simulink model "VCMGCM1962020b_v2"  (R2020b)
settings: Solver=FixedStepDiscrete  StartTime=0.0  StopTime=10.0  FixedStep=0.005  RelTol=1e-3  EnableMultiTasking=on
PreLoadFcn:
  | try, model_open; catch, disp('Error occurred while executing model pre-load callback: model_open.m'); disp('Please assure that the MATLAB working directory is set to the model directory before opening.'); end
InitFcn:
  | try, model_open; catch, end
undefined symbols (not defined in the file): Bridge, GCM, H, raptor_get_param_eval, raptor_get_safe_string, raptor_xcp_function
libraries: Blocks_lib x1165, Raptor_lib x665, simulink x62, VCM_lib x5
(part 20 of 23)

== system VCMGCM1962020b_v2/Fgnd/Virtual Sensors/Vehicle/Range/RangeGain/Subsystem ==
  y : Inport
  Enable : EnablePort
  Eqn(w/DvdByZeroPro) : Blocks_lib/Eqn(w//DvdByZeroPro)  eqn='u(1) / u(2)'  dmn='u(2)'  dfltval=0
  Out1 : Outport
  wires:
  y/1 -> Eqn(w/DvdByZeroPro)/1
  Eqn(w/DvdByZeroPro)/1 -> Out1/1

== system VCMGCM1962020b_v2/Fgnd/Actuators/CAN/Battery/ChgrBatt_State_Transition_Cmd/MsgTx/doublestrike ==
  note: Because of issues with the Romeo BMS this logic can be set up to apply main contactors followed by a reset and then contactor apply a second time
  <MainCntrReq [Bool]> : Inport
  AND{,2..4} (4 alike) : Logic  Operator=OR  AllPortsSameDT=off  OutDataTypeStr=boolean
  AND1 : Logic  AllPortsSameDT=off  OutDataTypeStr=boolean
  AND5 : Logic  AllPortsSameDT=off  OutDataTypeStr=boolean
  CntrSat1 : Blocks_lib/CntrSat  init=0  inc=1  typ=uint8  relop=>=  th_nam='MaincntrTurnOn'  th_gain=samptime  th_units='sec'  th_help='Counter threshold'  th_group='Group'
  CntrSat2 : Blocks_lib/CntrSat  init=0  inc=1  typ=uint8  relop=>=  th_nam='MaincntrTurnOff'  th_gain=samptime  th_units='sec'  th_help='Counter threshold'  th_group='Group'
  Falling edge : Subsystem
  Header : Blocks_lib/Header  width=Landscape  addtext=''
  NOT : Logic  Operator=NOT  AllPortsSameDT=off  OutDataTypeStr=boolean
  NOT1 : Logic  Operator=NOT  AllPortsSameDT=off  OutDataTypeStr=boolean
  raptor_adjustment : Raptor_lib/Data Storage/raptor_adjustment  paramName='RomoBMS2Strike'  nameSource=Parameter  initValue=0  dataType=boolean  storage=Calibration  calDispType=Number  calEnum={'False', 'True'}  calGain=1.0  calOffset=0.0  calMax=inf  calMin=-inf  calFormat='-1'  calUnit='Bool'  calHelp=' set this to 1 to turn on Batt main contr double strike logic'  calAccess=1  calFunction='Actuator | Batt '  calDispHeaders=off  calColHeaders={'Col1' 'Col2' 'Col3'}  calRowHeaders={'Row1' 'Row2' 'Row3'}
      settings: SourceProductName=Raptor
  raptor_measurement : Raptor_lib/Data Storage/raptor_measurement  paramName='CntrTest1'  nameSource=Parameter  calDispType=Number  calEnum={'False', 'True'}  calGain=1.0  calOffset=0.0  calMax=inf  calMin=-inf  calFormat='-1'  calUnit='bool'  calHelp='contactor reset logic test'  calAccess=1  calFunction=' Actuator | BMSTest'  calVisible=on
      settings: SourceProductName=Raptor
  raptor_measurement1 : Raptor_lib/Data Storage/raptor_measurement  paramName='CntrTest2'  nameSource=Parameter  calDispType=Number  calEnum={'False', 'True'}  calGain=1.0  calOffset=0.0  calMax=inf  calMin=-inf  calFormat='-1'  calUnit='bool'  calHelp='contactor reset logic test'  calAccess=1  calFunction=' Actuator | BMSTest'  calVisible=on
      settings: SourceProductName=Raptor
  rising edge : Subsystem
  rising edge1 : Subsystem
  HiVolt_Bus_Connect_Cmd1 : Outport
  wires:
  <MainCntrReq [Bool]>/1 -> CntrSat2/1, AND5/1, AND1/2, Falling edge/1(In), rising edge/1(In)
  AND3/1 -> CntrSat1/2
  AND1/1 -> AND/2
  NOT/1 -> AND1/1
  rising edge/1(rising) -> AND2/1
  CntrSat1/1 -> AND/1, raptor_measurement1/1
  Falling edge/1(falling) -> AND3/2, AND2/2
  CntrSat2/1 -> rising edge1/1(In), NOT/1, raptor_measurement/1, CntrSat1/1
  rising edge1/1(rising) -> AND3/1
  AND2/1 -> CntrSat2/2
  AND4/1 -> HiVolt_Bus_Connect_Cmd1/1
  AND/1 -> AND4/1  "HiVolt_Bus_Connect_Cmd"
  AND5/1 -> AND4/2
  raptor_adjustment/1 -> NOT1/1
  NOT1/1 -> AND5/2

== system VCMGCM1962020b_v2/Fgnd/Actuators/CAN/CCS Interface/CCSEV_ChargeParameters1/MsgTx/EVEnergyRequest ==
  Data : Inport
  Bus Selector : BusSelector  OutputSignals=VirtualSensors.Batt.BattSOC [%]
  Fcn : Fcn  Expr=u(1) * (u(2) - u(3)) /100
  Header : Blocks_lib/Header  width=Portrait  addtext=''
  Meas&Ovrd : Blocks_lib/Meas&Ovrd  nam=[nam 'EVEnergyRequest']  name_source=Parameter  view_as=Number  enum_struct={}  gain=1  min=-inf  max=inf  precision=''  units='kWh'  help='CAN message value'  group=['Actuators | CAN | ' msgnam]
  Mux : Mux  Inputs=3
  raptor_data_read : Raptor_lib/Data Storage/raptor_data_read  dataName=[nam 'FullSOC']  dataShape=Scalar  idxSource=Input  idxRow=1  idxCol=1
      settings: SourceProductName=Raptor
  raptor_data_read2 : Raptor_lib/Data Storage/raptor_data_read  dataName=[nam 'EnergyCapacity']  dataShape=Scalar  idxSource=Input  idxRow=1  idxCol=1
      settings: SourceProductName=Raptor
  kWh : Outport  VectorParamsAs1DForOutWhenUnconnected=off
  wires:
  Fcn/1 -> Meas&Ovrd/1
  Meas&Ovrd/1 -> kWh/1
  Bus Selector/1 -> Mux/3  "<BattSOC [%]>"
  Mux/1 -> Fcn/1
  raptor_data_read2/1 -> Mux/1
  raptor_data_read/1 -> Mux/2
  Data/1 -> Bus Selector/1

== system VCMGCM1962020b_v2/Fgnd/Actuators/CAN/CCS Interface/CCSEV_DC_ChargeInfo1/MsgTx/RemainingTime ==
  Data : Inport
  Bus Selector : BusSelector  OutputSignals=VirtualSensors.Batt.BattSOC [%],VirtualSensors.Batt.BattVolt [V],VirtualSensors.Batt.BattCur [A]
  Compare To Zero : simulink/Logic and Bit Operations/Compare To Zero  relop=<=  OutDataTypeStr=boolean
  Constant : Constant  Value=double(0)
  Demux : Demux  Outputs=2
  Eqn(w/DvdByZeroPro) : Blocks_lib/Eqn(w//DvdByZeroPro)  eqn='- u(1) * (u(2) - u(4)) / (u(5) * u(6)) * 600'  dmn='(u(5) * u(6))'  dfltval=127.5
  Eqn(w/DvdByZeroPro)1 : Blocks_lib/Eqn(w//DvdByZeroPro)  eqn='- u(1) * (u(3) - u(4)) / (u(5) * u(6)) * 600'  dmn='(u(5) * u(6))'  dfltval=127.5
  Fcn : Fcn  Expr=u(2) - u(4)
  Fcn1 : Fcn  Expr=u(3) - u(4)
  Filt : Blocks_lib/Filt  nam=[nam 'RemainingTimeFiltTC']  group=['Actuators | CAN | ' msgnam]  samptime=samptime
  Header : Blocks_lib/Header  width=Portrait  addtext=''
  Meas&Ovrd : Blocks_lib/Meas&Ovrd  nam=[nam 'RemainingTimeToFullSOC']  name_source=Parameter  view_as=Number  enum_struct={}  gain=1  min=-inf  max=inf  precision=''  units='minutes'  help='CAN message value'  group=['Actuators | CAN | ' msgnam]
  Meas&Ovrd1 : Blocks_lib/Meas&Ovrd  nam=[nam 'RemainingTimeToBulkSOC']  name_source=Parameter  view_as=Number  enum_struct={}  gain=1  min=-inf  max=inf  precision=''  units='minutes'  help='CAN message value'  group=['Actuators | CAN | ' msgnam]
  Multiport Switch : MultiPortSwitch  DataPortOrder=Zero-based contiguous  Inputs=2  zeroidx=on
  Mux : Mux  Inputs=6
  Mux1 : Mux  Inputs=2
  Mux2 : Mux  Inputs=2
  Saturation : Saturate  UpperLimit=0  LowerLimit=-inf
  Saturation1 : Saturate  UpperLimit=127.5  LowerLimit=0
  raptor_data_read : Raptor_lib/Data Storage/raptor_data_read  dataName=[nam 'FullSOC']  dataShape=Scalar  idxSource=Input  idxRow=1  idxCol=1
      settings: SourceProductName=Raptor
  raptor_data_read1 : Raptor_lib/Data Storage/raptor_data_read  dataName=[nam 'BulkSOC']  dataShape=Scalar  idxSource=Input  idxRow=1  idxCol=1
      settings: SourceProductName=Raptor
  raptor_data_read2 : Raptor_lib/Data Storage/raptor_data_read  dataName=[nam 'EnergyCapacity']  dataShape=Scalar  idxSource=Input  idxRow=1  idxCol=1
      settings: SourceProductName=Raptor
  Full : Outport  VectorParamsAs1DForOutWhenUnconnected=off
  Bulk : Outport  Port=2  VectorParamsAs1DForOutWhenUnconnected=off
  wires:
  Mux/1 -> Eqn(w/DvdByZeroPro)1/1, Eqn(w/DvdByZeroPro)/1, Fcn1/1, Fcn/1
  raptor_data_read1/1 -> Mux/3
  raptor_data_read/1 -> Mux/2
  Bus Selector/3 -> Saturation/1  "<BattCur [A]>"
  Bus Selector/2 -> Mux/5  "<BattVolt [V]>"
  Bus Selector/1 -> Mux/4  "<BattSOC [%]>"
  Meas&Ovrd1/1 -> Bulk/1
  raptor_data_read2/1 -> Mux/1
  Data/1 -> Bus Selector/1
  Meas&Ovrd/1 -> Full/1
  Saturation/1 -> Mux/6
  Eqn(w/DvdByZeroPro)/1 -> Mux1/1
  Eqn(w/DvdByZeroPro)1/1 -> Mux1/2
  Fcn/1 -> Mux2/1
  Fcn1/1 -> Mux2/2
  Mux2/1 -> Compare To Zero/1
  Compare To Zero/1 -> Multiport Switch/1
  Mux1/1 -> Multiport Switch/2
  Constant/1 -> Multiport Switch/3
  Saturation1/1 -> Filt/1
  Demux/1 -> Meas&Ovrd/1
  Demux/2 -> Meas&Ovrd1/1
  Filt/1 -> Demux/1
  Multiport Switch/1 -> Saturation1/1

== system VCMGCM1962020b_v2/Fgnd/Actuators/CAN/CCS Interface/Commands/Charge Port DC Voltage Diag/EvalDiag ==
  Data : Inport
  Reset : EnablePort  StatesWhenEnabling=reset
  Bus Selector : BusSelector  OutputSignals=VirtualSensors.Chgr.ChgPortDCVolt [V]
  FltRngTmr : Blocks_lib/FltRngTmr  nam='ChgPortDCVoltHi'  relop=>  threshnam='ChgPortDCVoltHiThr'  typ=double  units='V'  help='Range high fault threshold'  tmrth_nam='ChgPortDCVoltHiTimeThr'  tmrth_typ=uint16  tmrth_help='Range high fault time threshold'  samptime=samptime  group='Diagnostics | System'
  Header : Blocks_lib/Header  width=Portrait  addtext=''
  wires:
  Bus Selector/1 -> FltRngTmr/1  "<ChgPortDCVolt [V]>"
  Data/1 -> Bus Selector/1

== system VCMGCM1962020b_v2/Fgnd/Actuators/CAN/Charger/Config Msgs/Config Sequence/0x616 ==
  f : TriggerPort  TriggerType=function-call  VariantControl=Variant  PortDimensions=1
  Constant : Constant  Value=uint8(hex2dec('A5'))
  Header : Blocks_lib/Header  width=Portrait  addtext=''
  Logical Operator : Logic  Inputs=1  AllPortsSameDT=off  OutDataTypeStr=boolean
  Mux : Mux  Inputs=2
  Relational Operator : RelationalOperator  Operator===  OutDataTypeStr=boolean  RndMeth=Simplest
  Terminator : Terminator
  Terminator1 : Terminator
  Terminator2 : Terminator
  raptor_adjustment : Raptor_lib/Data Storage/raptor_adjustment  paramName='ChgrConfigData'  nameSource=Parameter  initValue=zeros(1,7)  dataType=uint8  storage=Calibration  calDispType=Number  calEnum={'False', 'True'}  calGain=1  calOffset=0  calMax=inf  calMin=-inf  calFormat=''  calUnit=''  calHelp='Charger configuration data'  calAccess=1  calFunction='Actuators | CAN | ChgrConfig'  calDispHeaders=off  calColHeaders={'Col1' 'Col2' 'Col3'}  calRowHeaders={'Row1' 'Row2' 'Row3'}
      settings: SourceProductName=Raptor
  raptor_can_rxraw : Raptor_lib/CAN/raptor_can_rxraw  canBus=bus  extendedId=0  showAge=0  id=hex2dec('616')  idMask=hex2dec('7FF')  mailbox='Chgr616Msg'  queueSize=1
      settings: SourceProductName=Raptor
  raptor_data_def : Raptor_lib/Data Storage/raptor_data_def  dataName='ChgrConfigComplete'  initValue=0  dataType=boolean  storage=Volatile (RAM)  calVisible=on  calType=Measurement  calDispType=Number  calEnum={'False', 'True'}  calGain=1.0  calOffset=0  calMin=-inf  calMax=inf  calFormat='-1'  calUnit='Bool'  calHelp='Charger configuration complete'  calAccess=1  calFunction='Actuators | CAN | ChgrConfig'  calDispHeaders=off  calColHeaders={'Col1' 'Col2' 'Col3'}  calRowHeaders={'Row1' 'Row2' 'Row3'}
      settings: SourceProductName=Raptor
  raptor_data_write : Raptor_lib/Data Storage/raptor_data_write  dataName='ChgrConfigComplete'  dataShape=Scalar  idxSource=Input Port  idxRow=1  idxCol=1
      settings: SourceProductName=Raptor
  wires:
  raptor_can_rxraw/1 -> Terminator/1
  raptor_can_rxraw/2 -> Terminator1/1
  raptor_can_rxraw/3 -> Terminator2/1
  raptor_can_rxraw/4 -> Relational Operator/1
  Logical Operator/1 -> raptor_data_write/1
  raptor_adjustment/1 -> Mux/1
  Constant/1 -> Mux/2
  Mux/1 -> Relational Operator/2
  Relational Operator/1 -> Logical Operator/1

== system VCMGCM1962020b_v2/Fgnd/Actuators/CAN/Charger/Config Msgs/Config Sequence/0x617_00 ==
  f : TriggerPort  TriggerType=function-call  VariantControl=Variant  PortDimensions=1
  Constant : Constant  Value=boolean(0)
  Constant1 : Constant  Value=uint32(hex2dec('617'))
  Constant2 : Constant  Value=uint8(8)
  Constant4 : Constant  Value=uint8(hex2dec('00'))
  Header : Blocks_lib/Header  width=Portrait  addtext=''
  Mux : Mux  Inputs=2
  raptor_can_txraw : Raptor_lib/CAN/raptor_can_txraw  canBus=bus  queueSize=1  showIdTypePort=1  idTypeSelectValues=Standard|Extended  idTypeSelect=Standard
      settings: SourceProductName=Raptor
  raptor_data_read : Raptor_lib/Data Storage/raptor_data_read  dataName='ChgrConfigData'  dataShape=Vector  idxSource=Read Entire Vector/Matrix  idxRow=1  idxCol=1
      settings: SourceProductName=Raptor
  wires:
  Constant2/1 -> raptor_can_txraw/3
  Constant1/1 -> raptor_can_txraw/2
  Constant/1 -> raptor_can_txraw/1
  Constant4/1 -> Mux/2
  raptor_data_read/1 -> Mux/1
  Mux/1 -> raptor_can_txraw/4

== system VCMGCM1962020b_v2/Fgnd/Actuators/CAN/Charger/Config Msgs/Config Sequence/0x617_A5 ==
  f : TriggerPort  TriggerType=function-call  VariantControl=Variant  PortDimensions=1
  Constant : Constant  Value=boolean(0)
  Constant1 : Constant  Value=uint32(hex2dec('617'))
  Constant2 : Constant  Value=uint8(8)
  Constant4 : Constant  Value=uint8(hex2dec('A5'))
  Header : Blocks_lib/Header  width=Portrait  addtext=''
  Mux : Mux  Inputs=2
  raptor_can_txraw : Raptor_lib/CAN/raptor_can_txraw  canBus=bus  queueSize=1  showIdTypePort=1  idTypeSelectValues=Standard|Extended  idTypeSelect=Standard
      settings: SourceProductName=Raptor
  raptor_data_read : Raptor_lib/Data Storage/raptor_data_read  dataName='ChgrConfigData'  dataShape=Vector  idxSource=Read Entire Vector/Matrix  idxRow=1  idxCol=1
      settings: SourceProductName=Raptor
  wires:
  Constant/1 -> raptor_can_txraw/1
  Constant1/1 -> raptor_can_txraw/2
  Constant2/1 -> raptor_can_txraw/3
  Mux/1 -> raptor_can_txraw/4
  Constant4/1 -> Mux/2
  raptor_data_read/1 -> Mux/1

== system VCMGCM1962020b_v2/Fgnd/Actuators/CAN/Drive Inverter/NMT Trasition Command/Inverter Error Reset/rising edge2 ==
  <RunMode [Bool]> : Inport
  AND6 : Logic  AllPortsSameDT=off  OutDataTypeStr=boolean
  NOT1 : Logic  Operator=NOT  AllPortsSameDT=off  OutDataTypeStr=boolean
  Unit Delay : UnitDelay  SampleTime=-1  HasFrameUpgradeWarning=on
  rising : Outport
  wires:
  Unit Delay/1 -> AND6/1
  NOT1/1 -> AND6/2
  AND6/1 -> rising/1
  <RunMode [Bool]>/1 -> NOT1/1, Unit Delay/1

== system VCMGCM1962020b_v2/Fgnd/Actuators/CAN/Other/A//C Compressor/MsgName/MsgTx ==
  Data : Inport
  Enable : EnablePort
  Bus Selector : BusSelector  OutputSignals=Control.Other.ACC.ACCSpdReq [rpm],Sensors.Sensors.Volt.DRVPVolt.DRVPVolt [V]
  CANTxField : Blocks_lib/CANTxField  custom=on  custom_nam=[nam '---']  custom_units='---'
  CANTxField1 : Blocks_lib/CANTxField  custom=on  custom_nam=[nam '---']  custom_units='---'
  Header : Blocks_lib/Header  width=Landscape  addtext=''
  Key Start : Subsystem
  raptor_can_txmsg : Raptor_lib/CAN/raptor_can_txmsg  canDefinition=struct('dbcFile', 'ACCompressor_MitsubishiEV36BNx.dbc','message', 'REQ','comment', '','signals', {{'SpdReq','BATT_VOLT','KeyStart'}},'enabled', [ 1 1 1;],'scaled', [ 1 1 1;],'canBus', 'bus','messageID', [ 202154048;],'idMask', [ 536870911;],'payloadMask', [],'payloadValue', [],'period', [ 100;],'mailbox', '''''','queueSize', [ 1;],'label', [ 1;],'ver', [ 2;],'showID', [ 0;],'showRaw', [ 0;],'fill', [ 1;],'editID', [ 0;],'signalOrder', [ 3;],'signalAscDes', [ 1;])  canBus=bus  queueSize=1  payloadMask=[]  payloadValue=[]  period=100  showID=0  label=1  idMask=hex2dec('1FFFFFFF')  fill=1  id=202154048  showRaw=0  signalOrder=3  signalInfo={{struct('Name', 'SpdReq','Startbit', [ 0;],'SignalSize', [ 14;],'ByteOrder', 'BigEndian','ValueType', 'UNSIGNED','Class', 'uint16','Signed', [ 0;],'Factor', [ 1;],'Offset', [ 0;],'Min', [ 960;],'Max', [ 8640;],'Units', 'RPM','Comment', '','StartBit', [ 8;]),struct('Name', 'BATT_VOLT','Startbit', [ 0;],'SignalSize', [ 8;],'ByteOrder', 'LittleEndian','ValueType', 'UNSIGNED','Class', 'uint8','Signed', [ 0;],'Factor', [ 0.1;],'Offset', [ 0;],'Min', [ 0;],'Max', [ 25.5;],'Units', 'Volts','Comment', '','StartBit', [ 24;]),struct('Name', 'KeyStart','Startbit', [ 0;],'SignalSize', [ 4;],'ByteOrder', 'LittleEndian','ValueType', 'UNSIGNED','Class', 'uint8','Signed', [ 0;],'Factor', [ 1;],'Offset', [ 0;],'Min', [ 0;],'Max', [ 3;],'Units', '','Comment', '','StartBit', [ 36;])}}
      settings: SourceProductName=Raptor
  wires:
  Data/1 -> Key Start/1(Data), Bus Selector/1
  CANTxField1/1 -> raptor_can_txmsg/2  "BATT_VOLT"
  Bus Selector/2 -> CANTxField1/1  "<DRVPVolt [V]>"
  Key Start/1(enum) -> raptor_can_txmsg/3  "KeyStart"
  CANTxField/1 -> raptor_can_txmsg/1  "SpdReq"
  Bus Selector/1 -> CANTxField/1  "<ACCSpdReq [rpm]>"

== system VCMGCM1962020b_v2/Fgnd/Actuators/CAN/Other/Cooling Pump 1/MsgName/MsgTx ==
  Data : Inport
  Enable : EnablePort
  Bus Selector : BusSelector  OutputSignals=Control.Other.CoolPump.CoolPump1EnblReq [Bool]
  Bus Selector1 : BusSelector  OutputSignals=Control.Other.CoolPump.CoolPump1SpdReq [%]
  CANTxField : Blocks_lib/CANTxField  custom=on  custom_nam=[nam '---']  custom_units='---'
  CANTxField1 : Blocks_lib/CANTxField  custom=on  custom_nam=[nam '---']  custom_units='---'
  Data Type Conversion : DataTypeConversion  OutDataTypeStr=uint32
  Header : Blocks_lib/Header  width=Landscape  addtext=''
  Shift Arithmetic : ArithShift  BitShiftNumber=-8
  raptor_adjustment : Raptor_lib/Data Storage/raptor_adjustment  paramName=[nam 'PowerHold']  nameSource=Parameter  initValue=0.00  dataType=uint8  storage=Calibration  calDispType=Number  calEnum={'False', 'True'}  calGain=1.0  calOffset=0.0  calMax=inf  calMin=-inf  calFormat='-1'  calUnit=''  calHelp='Power hold'  calAccess=1  calFunction=['Actuators | CAN | ' msgnam]  calDispHeaders=off  calColHeaders={'Col1' 'Col2' 'Col3'}  calRowHeaders={'Row1' 'Row2' 'Row3'}
      settings: SourceProductName=Raptor
  raptor_can_txmsg : Raptor_lib/CAN/raptor_can_txmsg  canDefinition=struct('dbcFile', 'EMPMotorController.dbc','message', 'EAPMCPC','comment', '','signals', {{'EnableCommand','PowerHold','SpeedCommand','PercentSpeed'}},'enabled', [ 1 1 1 0;],'canBus', 'bus','messageID', [ 410648576;],'idMask', [ 536805631;],'payloadMask', [],'payloadValue', [],'period', [ 1000;],'mailbox', '''''','queueSize', [ 1;],'label', [ 1;],'ver', [ 2;],'showID', [ 1;],'showRaw', [ 0;],'fill', [ 1;],'editID', [ 0;],'signalOrder', [ 3;])  canBus=bus  queueSize=1  payloadMask=[]  payloadValue=[]  period=1000  showID=1  label=1  idMask=hex2dec('1FFF00FF')  fill=1  id=410648576  showRaw=0  signalOrder=3  signalInfo={{struct('Name', 'EnableCommand','Startbit', [ 0;],'SignalSize', [ 2;],'ByteOrder', 'LittleEndian','ValueType', 'UNSIGNED','Class', 'uint8','Signed', [ 0;],'Factor', [ 1;],'Offset', [ 0;],'Min', [ 0;],'Max', [ 3;],'Units', '','Comment', '','StartBit', [ 0;]),struct('Name', 'PowerHold','Startbit', [ 0;],'SignalSize', [ 2;],'ByteOrder', 'LittleEndian','ValueType', 'UNSIGNED','Class', 'uint8','Signed', [ 0;],'Factor', [ 1;],'Offset', [ 0;],'Min', [ 0;],'Max', [ 3;],'Units', '','Comment', '','StartBit', [ 2;]),struct('Name', 'SpeedCommand','Startbit', [ 0;],'SignalSize', [ 16;],'ByteOrder', 'LittleEndian','ValueType', 'UNSIGNED','Class', 'uint16','Signed', [ 0;],'Factor', [ 0.5;],'Offset', [ 0;],'Min', [ 0;],'Max', [ 32127.5;],'Units', 'rpm','Comment', '','StartBit', [ 8;]),struct('Name', 'PercentSpeed','Startbit', [ 0;],'SignalSize', [ 8;],'ByteOrder', 'LittleEndian','ValueType', 'UNSIGNED','Class', 'uint8','Signed', [ 0;],'Factor', [ 0.5;],'Offset', [ 0;],'Min', [ 0;],'Max', [ 125;],'Units', '%','Comment', '','StartBit', [ 24;])}}
      settings: SourceProductName=Raptor
  raptor_data_read : Raptor_lib/Data Storage/raptor_data_read  dataName=[nam 'J1939SA']  dataShape=Scalar  idxSource=Input  idxRow=1  idxCol=1
      settings: SourceProductName=Raptor
  wires:
  Shift Arithmetic/1 -> raptor_can_txmsg/1
  raptor_data_read/1 -> Data Type Conversion/1
  Data Type Conversion/1 -> Shift Arithmetic/1
  raptor_adjustment/1 -> raptor_can_txmsg/3  "PowerHold"
  CANTxField1/1 -> raptor_can_txmsg/4  "SpeedCommand"
  Bus Selector1/1 -> CANTxField1/1  "<CoolPump1SpdReq [%]>"
  Bus Selector/1 -> CANTxField/1  "<CoolPump1EnblReq [Bool]>"
  CANTxField/1 -> raptor_can_txmsg/2  "EnableCommand"
  Data/1 -> Bus Selector/1, Bus Selector1/1

== system VCMGCM1962020b_v2/Fgnd/Actuators/CAN/Other/Cooling Pump 2/MsgName/MsgTx ==
  Data : Inport
  Enable : EnablePort
  Bus Selector : BusSelector  OutputSignals=Control.Other.CoolPump.CoolPump2EnblReq [Bool]
  Bus Selector1 : BusSelector  OutputSignals=Control.Other.CoolPump.CoolPump2SpdReq [%]
  CANTxField : Blocks_lib/CANTxField  custom=on  custom_nam=[nam '---']  custom_units='---'
  CANTxField1 : Blocks_lib/CANTxField  custom=on  custom_nam=[nam '---']  custom_units='---'
  Data Type Conversion : DataTypeConversion  OutDataTypeStr=uint32
  Header : Blocks_lib/Header  width=Landscape  addtext=''
  Shift Arithmetic : ArithShift  BitShiftNumber=-8
  raptor_adjustment : Raptor_lib/Data Storage/raptor_adjustment  paramName=[nam 'PowerHold']  nameSource=Parameter  initValue=0.00  dataType=uint8  storage=Calibration  calDispType=Number  calEnum={'False', 'True'}  calGain=1.0  calOffset=0.0  calMax=inf  calMin=-inf  calFormat='-1'  calUnit=''  calHelp='Power hold'  calAccess=1  calFunction=['Actuators | CAN | ' msgnam]  calDispHeaders=off  calColHeaders={'Col1' 'Col2' 'Col3'}  calRowHeaders={'Row1' 'Row2' 'Row3'}
      settings: SourceProductName=Raptor
  raptor_can_txmsg : Raptor_lib/CAN/raptor_can_txmsg  canDefinition=struct('dbcFile', 'EMPMotorController.dbc','message', 'EAPMCPC','comment', '','signals', {{'EnableCommand','PowerHold','SpeedCommand','PercentSpeed'}},'enabled', [ 1 1 1 0;],'canBus', 'bus','messageID', [ 410648576;],'idMask', [ 536805631;],'payloadMask', [],'payloadValue', [],'period', [ 1000;],'mailbox', '''''','queueSize', [ 1;],'label', [ 1;],'ver', [ 2;],'showID', [ 1;],'showRaw', [ 0;],'fill', [ 1;],'editID', [ 0;],'signalOrder', [ 3;])  canBus=bus  queueSize=1  payloadMask=[]  payloadValue=[]  period=1000  showID=1  label=1  idMask=hex2dec('1FFF00FF')  fill=1  id=410648576  showRaw=0  signalOrder=3  signalInfo={{struct('Name', 'EnableCommand','Startbit', [ 0;],'SignalSize', [ 2;],'ByteOrder', 'LittleEndian','ValueType', 'UNSIGNED','Class', 'uint8','Signed', [ 0;],'Factor', [ 1;],'Offset', [ 0;],'Min', [ 0;],'Max', [ 3;],'Units', '','Comment', '','StartBit', [ 0;]),struct('Name', 'PowerHold','Startbit', [ 0;],'SignalSize', [ 2;],'ByteOrder', 'LittleEndian','ValueType', 'UNSIGNED','Class', 'uint8','Signed', [ 0;],'Factor', [ 1;],'Offset', [ 0;],'Min', [ 0;],'Max', [ 3;],'Units', '','Comment', '','StartBit', [ 2;]),struct('Name', 'SpeedCommand','Startbit', [ 0;],'SignalSize', [ 16;],'ByteOrder', 'LittleEndian','ValueType', 'UNSIGNED','Class', 'uint16','Signed', [ 0;],'Factor', [ 0.5;],'Offset', [ 0;],'Min', [ 0;],'Max', [ 32127.5;],'Units', 'rpm','Comment', '','StartBit', [ 8;]),struct('Name', 'PercentSpeed','Startbit', [ 0;],'SignalSize', [ 8;],'ByteOrder', 'LittleEndian','ValueType', 'UNSIGNED','Class', 'uint8','Signed', [ 0;],'Factor', [ 0.5;],'Offset', [ 0;],'Min', [ 0;],'Max', [ 125;],'Units', '%','Comment', '','StartBit', [ 24;])}}
      settings: SourceProductName=Raptor
  raptor_data_read : Raptor_lib/Data Storage/raptor_data_read  dataName=[nam 'J1939SA']  dataShape=Scalar  idxSource=Input  idxRow=1  idxCol=1
      settings: SourceProductName=Raptor
  wires:
  Data/1 -> Bus Selector1/1, Bus Selector/1
  CANTxField/1 -> raptor_can_txmsg/2  "EnableCommand"
  Bus Selector/1 -> CANTxField/1  "<CoolPump2EnblReq [Bool]>"
  Bus Selector1/1 -> CANTxField1/1  "<CoolPump2SpdReq [%]>"
  CANTxField1/1 -> raptor_can_txmsg/4  "SpeedCommand"
  raptor_adjustment/1 -> raptor_can_txmsg/3  "PowerHold"
  Data Type Conversion/1 -> Shift Arithmetic/1
  raptor_data_read/1 -> Data Type Conversion/1
  Shift Arithmetic/1 -> raptor_can_txmsg/1

== system VCMGCM1962020b_v2/Fgnd/Actuators/CAN/Other/Heater/MsgName/MsgTx ==
  Data : Inport
  Enable : EnablePort
  Bus Selector : BusSelector  OutputSignals=Control.Other.Heater.HeaterOutletTempReq [degC]
  Bus Selector1 : BusSelector  OutputSignals=Control.Other.Heater.HeaterEnblReq [Bool]
  CANTxField : Blocks_lib/CANTxField  custom=off  custom_nam='---'  custom_units='---'
  CANTxField1 : Blocks_lib/CANTxField  custom=off  custom_nam='---'  custom_units='---'
  Header : Blocks_lib/Header  width=Landscape  addtext=''
  raptor_adjustment : Raptor_lib/Data Storage/raptor_adjustment  paramName='HTR_PWR_LIMIT'  nameSource=Parameter  initValue=0  dataType=double  storage=Calibration  calDispType=Number  calEnum={'False', 'True'}  calGain=1.0  calOffset=0.0  calMax=inf  calMin=-inf  calFormat='-1'  calUnit='W'  calHelp='Heater power limit'  calAccess=1  calFunction=['Actuators | CAN | ' msgnam]  calDispHeaders=off  calColHeaders={'Col1' 'Col2' 'Col3'}  calRowHeaders={'Row1' 'Row2' 'Row3'}
      settings: SourceProductName=Raptor
  raptor_adjustment1 : Raptor_lib/Data Storage/raptor_adjustment  paramName='ECU_MODE'  nameSource=Parameter  initValue=0  dataType=uint8  storage=Calibration  calDispType=Number  calEnum={'False', 'True'}  calGain=1.0  calOffset=0.0  calMax=inf  calMin=-inf  calFormat='-1'  calUnit=''  calHelp='ECU mode'  calAccess=1  calFunction=['Actuators | CAN | ' msgnam]  calDispHeaders=off  calColHeaders={'Col1' 'Col2' 'Col3'}  calRowHeaders={'Row1' 'Row2' 'Row3'}
      settings: SourceProductName=Raptor
  raptor_can_txmsg : Raptor_lib/CAN/raptor_can_txmsg  canDefinition=struct('dbcFile', 'ATSS17002_EWH40Dx-245.dbc','message', 'Data_Set_1','comment', '','signals', {{'HTR_OUTPUT_REQ','HTR_PWR_LIMIT','ECU_MODE','HTR_ENABLE'}},'enabled', [ 1 1 1 1;],'canBus', 'bus','messageID', [ 972;],'idMask', [ 536870911;],'payloadMask', [],'payloadValue', [],'period', [ 100;],'mailbox', '''''','queueSize', [ 1;],'label', [ 1;],'ver', [ 2;],'showID', [ 0;],'showRaw', [ 0;],'fill', [ 1;],'editID', [ 0;],'signalOrder', [ 3;])  canBus=bus  queueSize=1  payloadMask=[]  payloadValue=[]  period=100  showID=0  label=1  idMask=hex2dec('1FFFFFFF')  fill=1  id=972  showRaw=0  signalOrder=3  signalInfo={{struct('Name', 'HTR_OUTPUT_REQ','Startbit', [ 0;],'SignalSize', [ 8;],'ByteOrder', 'BigEndian','ValueType', 'UNSIGNED','Class', 'uint8','Signed', [ 0;],'Factor', [ 1;],'Offset', [ 0;],'Min', [ 0;],'Max', [ 80;],'Units', 'degC','Comment', 'Heater Output Request','StartBit', [ 0;]),struct('Name', 'HTR_PWR_LIMIT','Startbit', [ 0;],'SignalSize', [ 8;],'ByteOrder', 'BigEndian','ValueType', 'UNSIGNED','Class', 'uint8','Signed', [ 0;],'Factor', [ 40;],'Offset', [ 0;],'Min', [ 0;],'Max', [ 10160;],'Units', 'W','Comment', 'Heater Power Limit','StartBit', [ 8;]),struct('Name', 'ECU_MODE','Startbit', [ 0;],'SignalSize', [ 4;],'ByteOrder', 'BigEndian','ValueType', 'UNSIGNED','Class', 'uint8','Signed', [ 0;],'Factor', [ 1;],'Offset', [ 0;],'Min', [ 0;],'Max', [ 15;],'Units', '','Comment', 'Power Status Signal','StartBit', [ 16;]),struct('Name', 'HTR_ENABLE','Startbit', [ 0;],'SignalSize', [ 1;],'ByteOrder', 'BigEndian','ValueType', 'UNSIGNED','Class', 'uint8','Signed', [ 0;],'Factor', [ 1;],'Offset', [ 0;],'Min', [ 0;],'Max', [ 1;],'Units', '','Comment', 'Heater Enable/Disable','StartBit', [ 20;])}}
      settings: SourceProductName=Raptor
  wires:
  CANTxField/1 -> raptor_can_txmsg/1  "HTR_OUTPUT_REQ"
  Bus Selector/1 -> CANTxField/1  "<HeaterOutletTempReq [degC]>"
  raptor_adjustment/1 -> raptor_can_txmsg/2  "HTR_PWR_LIMIT"
  raptor_adjustment1/1 -> raptor_can_txmsg/3  "ECU_MODE"
  Bus Selector1/1 -> CANTxField1/1  "<HeaterEnblReq [Bool]>"
  CANTxField1/1 -> raptor_can_txmsg/4  "HTR_ENABLE"
  Data/1 -> Bus Selector/1, Bus Selector1/1

== system VCMGCM1962020b_v2/Fgnd/Actuators/CAN/Other/MPDM/MsgName/MsgTx ==
  Data : Inport
  Enable : EnablePort
  Bus Selector : BusSelector  OutputSignals=Control.Other.Other.SysWake [Bool],Control.Other.PrkPawl [Bool],Control.Other.BrkVacuumPump [Bool],Control.Other.Heater.HeaterPump [Bool],Control.Other.CoolFan [Bool]
  Constant : Constant  Value=uint8(hex2dec('80'))
  Constant1 : Constant  Value=uint8(0)
  Constant2 : Constant  Value=boolean(0)
  Data Type Conversion : DataTypeConversion  OutDataTypeStr=uint32
  Header : Blocks_lib/Header  width=Landscape  addtext=''
  Meas&Ovrd : Blocks_lib/Meas&Ovrd  nam='SysWake'  name_source=Parameter  view_as=Number  enum_struct={}  gain=1  min=-inf  max=inf  precision=''  units='Bool'  help='CAN field tx'  group=['Actuators | CAN | ' msgnam]
  Meas&Ovrd1 : Blocks_lib/Meas&Ovrd  nam='PrkPawl'  name_source=Parameter  view_as=Number  enum_struct={}  gain=1  min=-inf  max=inf  precision=''  units='Bool'  help='CAN field tx'  group=['Actuators | CAN | ' msgnam]
  Meas&Ovrd2 : Blocks_lib/Meas&Ovrd  nam='BrkVacuumPump'  name_source=Parameter  view_as=Number  enum_struct={}  gain=1  min=-inf  max=inf  precision=''  units='Bool'  help='CAN field tx'  group=['Actuators | CAN | ' msgnam]
  Meas&Ovrd3 : Blocks_lib/Meas&Ovrd  nam='HeaterPump'  name_source=Parameter  view_as=Number  enum_struct={}  gain=1  min=-inf  max=inf  precision=''  units='Bool'  help='CAN field tx'  group=['Actuators | CAN | ' msgnam]
  Meas&Ovrd4 : Blocks_lib/Meas&Ovrd  nam='CoolFan'  name_source=Parameter  view_as=Number  enum_struct={}  gain=1  min=-inf  max=inf  precision=''  units='Bool'  help='CAN field tx'  group=['Actuators | CAN | ' msgnam]
  Shift Arithmetic : ArithShift  BitShiftNumber=-8
  raptor_can_txmsg : Raptor_lib/CAN/raptor_can_txmsg  canDefinition=struct('dbcFile', 'MPDM.dbc','message', 'RelayCommand','comment', '','signals', {{'MessageID','GridAddress','Relay1','Relay2','Relay3','Relay4','Relay5','Relay6','Relay7','Relay8'}},'enabled', [ 1 1 1 1 1 1 1 1 1 1;],'canBus', 'bus','messageID', [ 418316288;],'idMask', [ 536805631;],'payloadMask', [],'payloadValue', [],'period', [ 100;],'mailbox', '','queueSize', [ 1;],'label', [ 0;],'ver', [ 2;],'showID', [ 1;],'showRaw', [ 0;],'fill', [ 0;],'editID', [ 0;],'signalOrder', [ 3;])  canBus=bus  queueSize=1  payloadMask=[]  payloadValue=[]  period=100  showID=1  label=0  idMask=hex2dec('1FFF00FF')  fill=0  id=418316288  showRaw=0  signalOrder=3  signalInfo={{struct('Name', 'MessageID','Startbit', [ 0;],'SignalSize', [ 8;],'ByteOrder', 'BigEndian','ValueType', 'UNSIGNED','Class', 'uint8','Signed', [ 0;],'Factor', [ 1;],'Offset', [ 0;],'Min', [ 0;],'Max', [ 255;],'Units', '','Comment', '','StartBit', [ 0;]),struct('Name', 'GridAddress','Startbit', [ 0;],'SignalSize', [ 8;],'ByteOrder', 'BigEndian','ValueType', 'UNSIGNED','Class', 'uint8','Signed', [ 0;],'Factor', [ 1;],'Offset', [ 0;],'Min', [ 0;],'Max', [ 255;],'Units', '','Comment', '','StartBit', [ 8;]),struct('Name', 'Relay1','Startbit', [ 0;],'SignalSize', [ 2;],'ByteOrder', 'BigEndian','ValueType', 'UNSIGNED','Class', 'uint8','Signed', [ 0;],'Factor', [ 1;],'Offset', [ 0;],'Min', [ 0;],'Max', [ 0;],'Units', '','Comment', '','StartBit', [ 16;]),struct('Name', 'Relay2','Startbit', [ 0;],'SignalSize', [ 2;],'ByteOrder', 'BigEndian','ValueType', 'UNSIGNED','Class', 'uint8','Signed', [ 0;],'Factor', [ 1;],'Offset', [ 0;],'Min', [ 0;],'Max', [ 0;],'Units', '','Comment', '','StartBit', [ 18;]),struct('Name', 'Relay3','Startbit', [ 0;],'SignalSize', [ 2;],'ByteOrder', 'BigEndian','ValueType', 'UNSIGNED','Class', 'uint8','Signed', [ 0;],'Factor', [ 1;],'Offset', [ 0;],'Min', [ 0;],'Max', [ 0;],'Units', '','Comment', '','StartBit', [ 20;]),struct('Name', 'Relay4','Startbit', [ 0;],'SignalSize', [ 2;],'ByteOrder', 'BigEndian','ValueType', 'UNSIGNED','Class', 'uint8','Signed', [ 0;],'Factor', [ 1;],'Offset', [ 0;],'Min', [ 0;],'Max', [ 0;],'Units', '','Comment', '','StartBit', [ 22;]),struct('Name', 'Relay5','Startbit', [ 0;],'SignalSize', [ 2;],'ByteOrder', 'BigEndian','ValueType', 'UNSIGNED','Class', 'uint8','Signed', [ 0;],'Factor', [ 1;],'Offset', [ 0;],'Min', [ 0;],'Max', [ 0;],'Units', '','Comment', '','StartBit', [ 24;]),struct('Name', 'Relay6','Startbit', [ 0;],'SignalSize', [ 2;],'ByteOrder', 'BigEndian','ValueType', 'UNSIGNED','Class', 'uint8','Signed', [ 0;],'Factor', [ 1;],'Offset', [ 0;],'Min', [ 0;],'Max', [ 0;],'Units', '','Comment', '','StartBit', [ 26;]),struct('Name', 'Relay7','Startbit', [ 0;],'SignalSize', [ 2;],'ByteOrder', 'BigEndian','ValueType', 'UNSIGNED','Class', 'uint8','Signed', [ 0;],'Factor', [ 1;],'Offset', [ 0;],'Min', [ 0;],'Max', [ 0;],'Units', '','Comment', '','StartBit', [ 28;]),struct('Name', 'Relay8','Startbit', [ 0;],'SignalSize', [ 2;],'ByteOrder', 'BigEndian','ValueType', 'UNSIGNED','Class', 'uint8','Signed', [ 0;],'Factor', [ 1;],'Offset', [ 0;],'Min', [ 0;],'Max', [ 0;],'Units', '','Comment', '','StartBit', [ 30;])}}
      settings: SourceProductName=Raptor
  raptor_data_read : Raptor_lib/Data Storage/raptor_data_read  dataName=[nam 'J1939SA']  dataShape=Scalar  idxSource=Input  idxRow=1  idxCol=1
      settings: SourceProductName=Raptor
  wires:
  raptor_data_read/1 -> Data Type Conversion/1
  Data Type Conversion/1 -> Shift Arithmetic/1
  Constant/1 -> raptor_can_txmsg/2
  Shift Arithmetic/1 -> raptor_can_txmsg/1
  Data/1 -> Bus Selector/1
  Constant1/1 -> raptor_can_txmsg/3
  Bus Selector/1 -> Meas&Ovrd/1  "<SysWake [Bool]>"
  Bus Selector/2 -> Meas&Ovrd1/1  "<PrkPawl [Bool]>"
  Bus Selector/3 -> Meas&Ovrd2/1  "<BrkVacuumPump [Bool]>"
  Bus Selector/4 -> Meas&Ovrd3/1  "<HeaterPump [Bool]>"
  Bus Selector/5 -> Meas&Ovrd4/1  "<CoolFan [Bool]>"
  Meas&Ovrd/1 -> raptor_can_txmsg/4
  Meas&Ovrd1/1 -> raptor_can_txmsg/5
  Meas&Ovrd2/1 -> raptor_can_txmsg/6
  Meas&Ovrd3/1 -> raptor_can_txmsg/7
  Meas&Ovrd4/1 -> raptor_can_txmsg/8
  Constant2/1 -> raptor_can_txmsg/9, raptor_can_txmsg/10, raptor_can_txmsg/11

== system VCMGCM1962020b_v2/Fgnd/Actuators/CAN/Other/Power Steering Pump Inverter/MsgName/MsgTx ==
  Data : Inport
  Enable : EnablePort
  Bus Selector : BusSelector  OutputSignals=Control.Other.PSPInvtr.PSPMtrSpdReq [rpm]
  CANTxField4 : Blocks_lib/CANTxField  custom=on  custom_nam=[nam 'SpeedLimitForward']  custom_units='---'
  Data Type Conversion : DataTypeConversion  OutDataTypeStr=uint32
  Gain : Gain  Gain=-1
  Header : Blocks_lib/Header  width=Landscape  addtext=''
  Shift Arithmetic : ArithShift  BitShiftNumber=-8
  raptor_adjustment1 : Raptor_lib/Data Storage/raptor_adjustment  paramName=[nam 'TorqueRegenLimit']  nameSource=Parameter  initValue=-10  dataType=double  storage=Calibration  calDispType=Number  calEnum={'Disabled', 'Enabled'}  calGain=1  calOffset=0  calMax=inf  calMin=-inf  calFormat=''  calUnit='Nm'  calHelp='Torque regeneration limit'  calAccess=1  calFunction=['Actuators | CAN | ' msgnam]  calDispHeaders=off  calColHeaders={'Col1' 'Col2' 'Col3'}  calRowHeaders={'Row1' 'Row2' 'Row3'}
      settings: SourceProductName=Raptor
  raptor_can_txmsg : Raptor_lib/CAN/raptor_can_txmsg  canDefinition=struct('dbcFile', 'SevconInverter_H_Protocol.dbc','message', 'HC2_Demands','comment', '','signals', {{'SEQ_Command2','CS_Command2','Speed_Limit_Reverse','Torque_Regen_Limit','Speed_Limit_Forward'}},'enabled', [ 0 0 1 1 1;],'canBus', 'bus','messageID', [ 420544767;],'idMask', [ 536805631;],'payloadMask', [],'payloadValue', [],'period', [ 100;],'mailbox', '''''','queueSize', [ 1;],'label', [ 1;],'ver', [ 2;],'showID', [ 1;],'showRaw', [ 0;],'fill', [ 0;],'editID', [ 1;],'signalOrder', [ 3;])  canBus=bus  queueSize=1  payloadMask=[]  payloadValue=[]  period=100  showID=1  label=1  idMask=hex2dec('1FFF00FF')  fill=0  id=420544767  showRaw=0  signalOrder=3  signalInfo={{struct('Name', 'SEQ_Command2','Startbit', [ 0;],'SignalSize', [ 8;],'ByteOrder', 'LittleEndian','ValueType', 'UNSIGNED','Class', 'uint8','Signed', [ 0;],'Factor', [ 1;],'Offset', [ 0;],'Min', [ 0;],'Max', [ 255;],'Units', '','Comment', '','StartBit', [ 48;]),struct('Name', 'CS_Command2','Startbit', [ 0;],'SignalSize', [ 8;],'ByteOrder', 'LittleEndian','ValueType', 'UNSIGNED','Class', 'uint8','Signed', [ 0;],'Factor', [ 1;],'Offset', [ 0;],'Min', [ 0;],'Max', [ 255;],'Units', '','Comment', '','StartBit', [ 56;]),struct('Name', 'Speed_Limit_Reverse','Startbit', [ 0;],'SignalSize', [ 16;],'ByteOrder', 'LittleEndian','ValueType', 'SIGNED','Class', 'int16','Signed', [ 1;],'Factor', [ 1;],'Offset', [ 0;],'Min', [ -32768;],'Max', [ 0;],'Units', 'RPM','Comment', '','StartBit', [ 32;]),struct('Name', 'Torque_Regen_Limit','Startbit', [ 0;],'SignalSize', [ 16;],'ByteOrder', 'LittleEndian','ValueType', 'SIGNED','Class', 'int16','Signed', [ 1;],'Factor', [ 0.0625;],'Offset', [ 0;],'Min', [ -2048;],'Max', [ 0;],'Units', 'Nm','Comment', '','StartBit', [ 0;]),struct('Name', 'Speed_Limit_Forward','Startbit', [ 0;],'SignalSize', [ 16;],'ByteOrder', 'LittleEndian','ValueType', 'SIGNED','Class', 'int16','Signed', [ 1;],'Factor', [ 1;],'Offset', [ 0;],'Min', [ 0;],'Max', [ 32767;],'Units', 'RPM','Comment', '','StartBit', [ 16;])}}
      settings: SourceProductName=Raptor
  raptor_data_read : Raptor_lib/Data Storage/raptor_data_read  dataName=[nam 'J1939SA']  dataShape=Scalar  idxSource=Input  idxRow=1  idxCol=1
      settings: SourceProductName=Raptor
  wires:
  Shift Arithmetic/1 -> raptor_can_txmsg/1
  Gain/1 -> raptor_can_txmsg/2  "Speed_Limit_Reverse"
  Bus Selector/1 -> CANTxField4/1  "<PSPMtrSpdReq [rpm]>"
  Data/1 -> Bus Selector/1
  raptor_adjustment1/1 -> raptor_can_txmsg/3  "Torque_Regen_Limit"
  Data Type Conversion/1 -> Shift Arithmetic/1
  raptor_data_read/1 -> Data Type Conversion/1
  CANTxField4/1 -> raptor_can_txmsg/4, Gain/1  "Speed_Limit_Forward"

== system VCMGCM1962020b_v2/Fgnd/Actuators/CAN/Other/Power Steering Pump Inverter/PSPInvtrHC1_Demands/MsgTx ==
  Data : Inport
  Enable : EnablePort
  Control Word : Subsystem
      settings: OpenFcn=open_system(gcb,'force')
  Data Type Conversion : DataTypeConversion  OutDataTypeStr=uint32
  Header : Blocks_lib/Header  width=Landscape  addtext=''
  Shift Arithmetic : ArithShift  BitShiftNumber=-8
  raptor_adjustment : Raptor_lib/Data Storage/raptor_adjustment  paramName=[nam 'TorqueTractionLimit']  nameSource=Parameter  initValue=10  dataType=double  storage=Calibration  calDispType=Number  calEnum={'Disabled', 'Enabled'}  calGain=1  calOffset=0  calMax=inf  calMin=-inf  calFormat=''  calUnit='Nm'  calHelp='Torque traction limit'  calAccess=1  calFunction=['Actuators | CAN | ' msgnam]  calDispHeaders=off  calColHeaders={'Col1' 'Col2' 'Col3'}  calRowHeaders={'Row1' 'Row2' 'Row3'}
      settings: SourceProductName=Raptor
  raptor_adjustment1 : Raptor_lib/Data Storage/raptor_adjustment  paramName=[nam 'TorqueRequest']  nameSource=Parameter  initValue=10  dataType=double  storage=Calibration  calDispType=Number  calEnum={'Disabled', 'Enabled'}  calGain=1  calOffset=0  calMax=inf  calMin=-inf  calFormat=''  calUnit='Nm'  calHelp='Torque request'  calAccess=1  calFunction=['Actuators | CAN | ' msgnam]  calDispHeaders=off  calColHeaders={'Col1' 'Col2' 'Col3'}  calRowHeaders={'Row1' 'Row2' 'Row3'}
      settings: SourceProductName=Raptor
  raptor_can_txmsg : Raptor_lib/CAN/raptor_can_txmsg  canDefinition=struct('dbcFile', 'SevconInverter_H_Protocol.dbc','message', 'HC1_Demands','comment', '','signals', {{'SEQ_Command1','CS_Command1','Torque_Traction_Limit','ControlWord','Torque_Request'}},'enabled', [ 0 0 1 1 1;],'canBus', 'bus','messageID', [ 420479231;],'idMask', [ 536805631;],'payloadMask', [],'payloadValue', [],'period', [ 100;],'mailbox', '''''','queueSize', [ 1;],'label', [ 1;],'ver', [ 2;],'showID', [ 1;],'showRaw', [ 0;],'fill', [ 0;],'editID', [ 1;],'signalOrder', [ 3;])  canBus=bus  queueSize=1  payloadMask=[]  payloadValue=[]  period=100  showID=1  label=1  idMask=hex2dec('1FFF00FF')  fill=0  id=420479231  showRaw=0  signalOrder=3  signalInfo={{struct('Name', 'SEQ_Command1','Startbit', [ 0;],'SignalSize', [ 8;],'ByteOrder', 'LittleEndian','ValueType', 'UNSIGNED','Class', 'uint8','Signed', [ 0;],'Factor', [ 1;],'Offset', [ 0;],'Min', [ 0;],'Max', [ 255;],'Units', '','Comment', '','StartBit', [ 48;]),struct('Name', 'CS_Command1','Startbit', [ 0;],'SignalSize', [ 8;],'ByteOrder', 'LittleEndian','ValueType', 'UNSIGNED','Class', 'uint8','Signed', [ 0;],'Factor', [ 1;],'Offset', [ 0;],'Min', [ 0;],'Max', [ 255;],'Units', '','Comment', '','StartBit', [ 56;]),struct('Name', 'Torque_Traction_Limit','Startbit', [ 0;],'SignalSize', [ 16;],'ByteOrder', 'LittleEndian','ValueType', 'SIGNED','Class', 'int16','Signed', [ 1;],'Factor', [ 0.0625;],'Offset', [ 0;],'Min', [ 0;],'Max', [ 2047.9375;],'Units', 'Nm','Comment', '','StartBit', [ 32;]),struct('Name', 'ControlWord','Startbit', [ 0;],'SignalSize', [ 16;],'ByteOrder', 'LittleEndian','ValueType', 'UNSIGNED','Class', 'uint16','Signed', [ 0;],'Factor', [ 1;],'Offset', [ 0;],'Min', [ 0;],'Max', [ 65535;],'Units', 'enum','Comment', '','StartBit', [ 16;]),struct('Name', 'Torque_Request','Startbit', [ 0;],'SignalSize', [ 16;],'ByteOrder', 'LittleEndian','ValueType', 'SIGNED','Class', 'int16','Signed', [ 1;],'Factor', [ 0.0625;],'Offset', [ 0;],'Min', [ -2048;],'Max', [ 2047.9375;],'Units', 'Nm','Comment', '','StartBit', [ 0;])}}
      settings: SourceProductName=Raptor
  raptor_data_read : Raptor_lib/Data Storage/raptor_data_read  dataName=[nam 'J1939SA']  dataShape=Scalar  idxSource=Input  idxRow=1  idxCol=1
      settings: SourceProductName=Raptor
  wires:
  Data/1 -> Control Word/1(Data)
  Control Word/1(enum) -> raptor_can_txmsg/3  "ControlWord"
  raptor_adjustment1/1 -> raptor_can_txmsg/4  "Torque_Request"
  raptor_adjustment/1 -> raptor_can_txmsg/2  "Torque_Traction_Limit"
  Shift Arithmetic/1 -> raptor_can_txmsg/1
  Data Type Conversion/1 -> Shift Arithmetic/1
  raptor_data_read/1 -> Data Type Conversion/1

== system VCMGCM1962020b_v2/Fgnd/Actuators/CAN/Other/Power Steering Pump Inverter/PSPInvtrHC3_Battery_Demands/MsgTx ==
  Data : Inport
  Enable : EnablePort
  Data Type Conversion : DataTypeConversion  OutDataTypeStr=uint32
  Header : Blocks_lib/Header  width=Landscape  addtext=''
  Shift Arithmetic : ArithShift  BitShiftNumber=-8
  Terminator : Terminator
  raptor_adjustment1 : Raptor_lib/Data Storage/raptor_adjustment  paramName=[nam 'LinkVoltageTarget']  nameSource=Parameter  initValue=0  dataType=double  storage=Calibration  calDispType=Number  calEnum={'Disabled', 'Enabled'}  calGain=1  calOffset=0  calMax=inf  calMin=-inf  calFormat=''  calUnit='V'  calHelp='Link voltage target'  calAccess=1  calFunction=['Actuators | CAN | ' msgnam]  calDispHeaders=off  calColHeaders={'Col1' 'Col2' 'Col3'}  calRowHeaders={'Row1' 'Row2' 'Row3'}
      settings: SourceProductName=Raptor
  raptor_adjustment2 : Raptor_lib/Data Storage/raptor_adjustment  paramName=[nam 'DCLinkImaxRecharge']  nameSource=Parameter  initValue=-10  dataType=double  storage=Calibration  calDispType=Number  calEnum={'Disabled', 'Enabled'}  calGain=1  calOffset=0  calMax=inf  calMin=-inf  calFormat=''  calUnit='A'  calHelp='DC link Imax recharge'  calAccess=1  calFunction=['Actuators | CAN | ' msgnam]  calDispHeaders=off  calColHeaders={'Col1' 'Col2' 'Col3'}  calRowHeaders={'Row1' 'Row2' 'Row3'}
      settings: SourceProductName=Raptor
  raptor_adjustment3 : Raptor_lib/Data Storage/raptor_adjustment  paramName=[nam 'DCLinkImaxDischarge']  nameSource=Parameter  initValue=10  dataType=double  storage=Calibration  calDispType=Number  calEnum={'Disabled', 'Enabled'}  calGain=1  calOffset=0  calMax=inf  calMin=-inf  calFormat=''  calUnit='A'  calHelp='DC link Imax discharge'  calAccess=1  calFunction=['Actuators | CAN | ' msgnam]  calDispHeaders=off  calColHeaders={'Col1' 'Col2' 'Col3'}  calRowHeaders={'Row1' 'Row2' 'Row3'}
      settings: SourceProductName=Raptor
  raptor_can_txmsg : Raptor_lib/CAN/raptor_can_txmsg  canDefinition=struct('dbcFile', 'SevconInverter_H_Protocol.dbc','message', 'HC3_Battery_Demands','comment', '','signals', {{'DC_Link_Voltage_Target','SEQ_CurrentLimits','CS_CurrentLimits','DC_Link_Imax_Recharge','DC_Link_Imax_Discharge'}},'enabled', [ 1 0 0 1 1;],'canBus', 'bus','messageID', [ 420610303;],'idMask', [ 536805631;],'payloadMask', [],'payloadValue', [],'period', [ 100;],'mailbox', '''''','queueSize', [ 1;],'label', [ 1;],'ver', [ 2;],'showID', [ 1;],'showRaw', [ 0;],'fill', [ 0;],'editID', [ 1;],'signalOrder', [ 3;])  canBus=bus  queueSize=1  payloadMask=[]  payloadValue=[]  period=100  showID=1  label=1  idMask=hex2dec('1FFF00FF')  fill=0  id=420610303  showRaw=0  signalOrder=3  signalInfo={{struct('Name', 'DC_Link_Voltage_Target','Startbit', [ 0;],'SignalSize', [ 16;],'ByteOrder', 'LittleEndian','ValueType', 'SIGNED','Class', 'int16','Signed', [ 1;],'Factor', [ 0.0625;],'Offset', [ 0;],'Min', [ 0;],'Max', [ 0;],'Units', 'V','Comment', '','StartBit', [ 32;]),struct('Name', 'SEQ_CurrentLimits','Startbit', [ 0;],'SignalSize', [ 8;],'ByteOrder', 'LittleEndian','ValueType', 'UNSIGNED','Class', 'uint8','Signed', [ 0;],'Factor', [ 1;],'Offset', [ 0;],'Min', [ 0;],'Max', [ 255;],'Units', '','Comment', '','StartBit', [ 48;]),struct('Name', 'CS_CurrentLimits','Startbit', [ 0;],'SignalSize', [ 8;],'ByteOrder', 'LittleEndian','ValueType', 'UNSIGNED','Class', 'uint8','Signed', [ 0;],'Factor', [ 1;],'Offset', [ 0;],'Min', [ 0;],'Max', [ 255;],'Units', '','Comment', '','StartBit', [ 56;]),struct('Name', 'DC_Link_Imax_Recharge','Startbit', [ 0;],'SignalSize', [ 16;],'ByteOrder', 'LittleEndian','ValueType', 'SIGNED','Class', 'int16','Signed', [ 1;],'Factor', [ 1;],'Offset', [ 0;],'Min', [ -1000;],'Max', [ 0;],'Units', 'A','Comment', '','StartBit', [ 16;]),struct('Name', 'DC_Link_Imax_Discharge','Startbit', [ 0;],'SignalSize', [ 16;],'ByteOrder', 'LittleEndian','ValueType', 'SIGNED','Class', 'int16','Signed', [ 1;],'Factor', [ 1;],'Offset', [ 0;],'Min', [ 0;],'Max', [ 1000;],'Units', 'A','Comment', '','StartBit', [ 0;])}}
      settings: SourceProductName=Raptor
  raptor_data_read : Raptor_lib/Data Storage/raptor_data_read  dataName=[nam 'J1939SA']  dataShape=Scalar  idxSource=Input  idxRow=1  idxCol=1
      settings: SourceProductName=Raptor
  wires:
  Shift Arithmetic/1 -> raptor_can_txmsg/1
  raptor_adjustment3/1 -> raptor_can_txmsg/4  "DC_Link_Imax_Discharge"
  raptor_adjustment1/1 -> raptor_can_txmsg/2  "DC_Link_Voltage_Target"
  Data/1 -> Terminator/1
  raptor_adjustment2/1 -> raptor_can_txmsg/3  "DC_Link_Imax_Recharge"
  Data Type Conversion/1 -> Shift Arithmetic/1
  raptor_data_read/1 -> Data Type Conversion/1

== system VCMGCM1962020b_v2/Fgnd/Control/Drive Inverter/Motor Torque Request/Driver Torque Request/Cruise Control/Control ==
  Data : Inport
  PedTrq : Inport  Port=2
  Setpt : Inport  Port=3
  Reset : EnablePort  StatesWhenEnabling=reset
  Add : Sum
  Arbitration State : Subsystem
  Bus Selector1 : BusSelector  OutputSignals=CCSetpt [kph]
  Bus Selector2 : BusSelector  OutputSignals=CCSetpt [kph]
  Bus Selector3 : BusSelector  OutputSignals=VirtualSensors.Spd.VehSpd [kph]
  Header : Blocks_lib/Header  width=Portrait  addtext=''
  Multiport Switch : MultiPortSwitch  DataPortOrder=Zero-based contiguous  Inputs=2  zeroidx=on
  PICtrl(w/VarGain)(w/ICInport)(w/AntiWindup) : Subsystem  mask{nam='CC', dim=9, inunits='kph', units='Nm', group=group, samptime=samptime}
      mask prompts: nam "Name"; dim "Gain Table Dimension"; inunits "Input Units"; units "Output Units"; samptime "Sample Time (sec)"
      mask Display: disp(['PI Control\n(w/ Variable Gain)\n(w/ IC Inport)\n(w/ AntiWindup)\n' nam]);
  "Reset, IC, & Limits" : Subsystem
  Unit Delay : UnitDelay  SampleTime=-1  HasFrameUpgradeWarning=on
  raptor_measurement1 : Raptor_lib/Data Storage/raptor_measurement  paramName='CCTrqReq'  nameSource=Parameter  calDispType=Number  calEnum={'Not adapting', 'Adapting'}  calGain=1  calOffset=0  calMax=inf  calMin=-inf  calFormat=''  calUnit='Nm'  calHelp='Cruise control torque request'  calAccess=1  calFunction=group  calVisible=on
      settings: SourceProductName=Raptor
  raptor_table_1d : Raptor_lib/Table Lookup/raptor_table_1d  dataName='CCFeedfwdTbl'  initValue=zeros(1,17)  dataType=double  storage=Calibration  initValueX=[1:17]  dataTypeXY=double  storageXY=Calibration  calVisible=on  showTable=on  calGain=1.0  calOffset=0.0  calMax=Inf  calMin=-Inf  calFormat='-1'  calUnit='Nm'  calHelp='Cruise control feedforward term'  showBreakpoint=on  dataNameX='CCSetpt17IdxArr'  calGainX=1.0  calOffsetX=0.0  calMaxX=Inf  calMinX=-Inf  calFormatX='-1'  calUnitX='kph'  calHelpX='Index array'  calAccess=1  calFunction=group  measureEnable=on  mName='CCFeedfwd'
      settings: SourceProductName=Raptor
  Nm : Outport  VectorParamsAs1DForOutWhenUnconnected=off
  wires:
  Multiport Switch/1 -> raptor_measurement1/1, Nm/1
  Bus Selector1/1 -> PICtrl(w/VarGain)(w/ICInport)(w/AntiWindup)/1(Setpt)  "<CCSetpt [kph]>"
  raptor_table_1d/1 -> "Reset, IC, & Limits"/3(FF), Add/1
  PICtrl(w/VarGain)(w/ICInport)(w/AntiWindup)/1(Cmd) -> Add/2
  Add/1 -> Multiport Switch/2, Unit Delay/1
  Bus Selector3/1 -> PICtrl(w/VarGain)(w/ICInport)(w/AntiWindup)/2(Act)  "<VehSpd [kph]>"
  Unit Delay/1 -> Arbitration State/2(PIReq)
  "Reset, IC, & Limits"/1(Rst) -> PICtrl(w/VarGain)(w/ICInport)(w/AntiWindup)/3(Rst)
  Arbitration State/1("PedWinArb ") -> Multiport Switch/1, "Reset, IC, & Limits"/4(PedWinArb)
  "Reset, IC, & Limits"/2(" IC ") -> PICtrl(w/VarGain)(w/ICInport)(w/AntiWindup)/4(IC)
  "Reset, IC, & Limits"/4(Mx) -> PICtrl(w/VarGain)(w/ICInport)(w/AntiWindup)/6(Mx)
  "Reset, IC, & Limits"/5(Mn) -> PICtrl(w/VarGain)(w/ICInport)(w/AntiWindup)/7(Mn)
  PedTrq/1 -> Arbitration State/1(PedTrq), Multiport Switch/3
  Setpt/1 -> Bus Selector2/1, "Reset, IC, & Limits"/2(Setpt), Bus Selector1/1
  Data/1 -> "Reset, IC, & Limits"/1(Data), Bus Selector3/1
  "Reset, IC, & Limits"/3(" Hold") -> PICtrl(w/VarGain)(w/ICInport)(w/AntiWindup)/5(Hold)
  Bus Selector2/1 -> raptor_table_1d/1  "<CCSetpt [kph]>"
